simulink model "VC_v1p1"  (R2022b)
settings: Solver=VariableStepAuto  StartTime=0.0  StopTime=inf  FixedStep=1/100  MaxStep=ts  RelTol=1e-3
InitFcn:
  | init_car
  | init_par
values from neighbouring files (symbols this model uses):
  east0 = EWP(1)    [run_VC_bench.m]
  g = 9.81    [init_car.m]
  north0 = NWP(1)    [run_VC_bench.m]
  NUM_WP = length(NWP)    [run_VC_bench.m]
  psi0 = (pi/180)*HWP(1)    [run_VC_bench.m]
  ts = 1/fs    (= 0.01)    [init_car.m]
  vcg0 = 0    [run_VC_bench.m]
  WPT_MTX = [NWP,EWP,HWP,VWP,KWP,SWP]    [run_VC_bench.m]
undefined symbols (not defined in the file or in its folder): car, EWP, NWP, par, ZWP
libraries: simulink x9, matrix_library x6
(part 1 of 3)
Description:
  | This simulation was created by S. C. Southward to develop and validate control strategies for an autonomous vehicle modeled as a kinematic bicycle model.
settings Model: Creator=steve  LastModifiedBy=steve
settings SolverCC: AlgebraicLoopSolver=TrustRegion
settings DataIOCC: SaveOutput=off  SignalLogging=off  DSMLogging=off  SaveTime=off  ReturnWorkspaceOutputs=off
settings OptimizationCC: DefaultParameterBehavior=Inlined  UseDivisionForNetSlopeComputation=on  GainParamInheritBuiltInType=on  UseFloatMulNetSlope=on  InlineInvariantSignals=on  PassReuseOutputArgsAs=Individual arguments  ZeroExternalMemoryAtStartup=off  ZeroInternalMemoryAtStartup=off  NoFixptDivByZeroProtection=on  EfficientFloat2IntCast=on  LifeSpan=1  OptimizeBlockOrder=speed  DifferentSizesBufferReuse=on  EfficientTunableParamExpr=on
settings DebuggingCC: MaxConsecutiveZCsMsg=none  ParameterTunabilityLossMsg=error  UnderSpecifiedDataTypeMsg=warning  UnconnectedInputMsg=warning  UnconnectedOutputMsg=warning  UnconnectedLineMsg=warning  SFMachineParentedDataDiag=warning  UnderSpecifiedDimensionMsg=warning  ArithmeticOperatorsInVariantConditions=warning
settings HardwareCC: ProdBitPerLong=64  ProdLongLongMode=on  ProdHWDeviceType=Intel->x86-64 (Linux 64)
settings ModelReferenceCC: EnableRefExpFcnMdlSchedulingChecks=on
settings SFSimCC: SimUseLocalCustomCode=off  MATLABDynamicMemAlloc=off  CustomCodeUndefinedFunction=UseInterfaceOnly
settings RTWCC: Description=Embedded Coder  SystemTargetFile=ert.tlc  TemplateMakefile=ert_default_tmf  RTWUseLocalCustomCode=off  TargetLang=C++  DLArmComputeVersion=19.05
settings CodeAppCC: ForceParamTrailComments=on  IgnoreCustomStorageClasses=off  OperatorAnnotations=on  SimulinkDataObjDesc=on  SFDataObjDesc=on  CustomSymbolStrGlobalVar=rt$N$M  CustomSymbolStrType=$N$M  CustomSymbolStrFcn=$N$M$F  CustomSymbolStrMacro=$N$M  InsertBlockDesc=on
settings ERTTargetCC: TargetLangStandard=C++03 (ISO)  GenerateSampleERTMain=on  IncludeMdlTerminateFcn=off  CombineSignalStateStructs=on  CodeInterfacePackaging=C++ class  SupportComplex=off  SupportNonInlinedSFcns=on  InlinedParameterPlacement=NonHierarchical  RootIOFormat=Structure reference  ERTCustomFileTemplate=example_file_process.tlc  ERTFilePackagingFormat=CompactWithDataFile

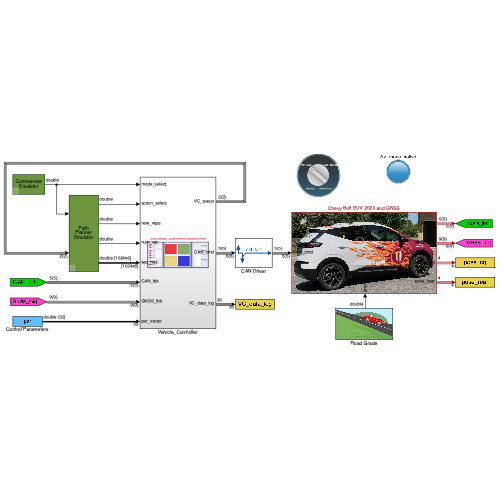
[thumbnail: Simulink's stored preview of the top-level diagram]
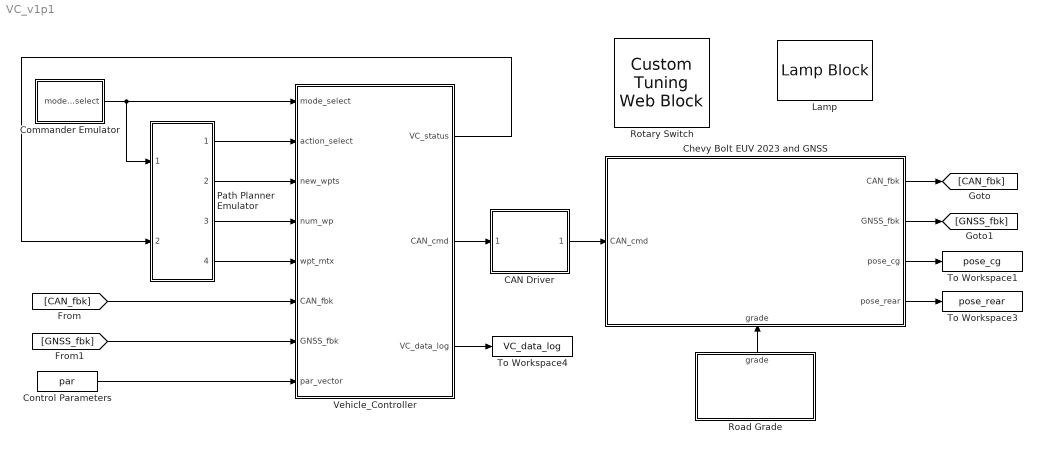
== system VC_v1p1 ==
  CAN Driver : Subsystem
      mask Display: image('$imagefile'); % Use "Edit Image" on toolstrip to change.
  Chevy Bolt EUV 2023 and GNSS : Subsystem
      settings: PortSchema="{\"entries\":[{\"content\":{\"sides\":[{\"content\":{\"connectorIds\":[\"In1\"]},\"type\":\"ConnectorPlacement.EquallySpacedRectSide\",\"uuid\":\"214ac55f-e1ad-4aeb-894e-d0c732f6c7ee\"},{\"content\":{\"connectorIds\":[\"Out1\",\"Out2\",\"Out3\",\"Out4\"],\"side\":\"RIGHT\"},\"type\":\"ConnectorPlacement.EquallySpacedRectSide\",\"uuid\":\"96b26d7b-3219-4372-aec8-5812d174b28b\"},{\"content\":{\"connectorIds\":[],\"side\":\"TOP\"},\"type\":\"ConnectorPlacement.EquallySpacedRectSide\",\"uuid\":\"1264bf6a-3e04-4574-8398-8e873a97a666\"},{\"content\":{\"connectorIds\":[\"In2\"],\"side\":\"BOTTOM\"},\"type\":\"ConnectorPlacement.EquallySpacedRectSide\",\"uuid\":\"d9b028eb-d70e-44ed-81e4-9460dc761106\"}]},\"type\":\"ConnectorPlacement.EquallySpacedConnector\",\"uuid\":\"c4360da5-3195-43cb-bf9a-daa7ef28b28e\"}],\"packageUris\":[\"http://schema.mathworks.com/mf0/Connector/R2020b\"],\"version\":\"1.0\"}"
      mask Display: image('$imagefile'); % Use "Edit Image" on toolstrip to change.
  Commander Emulator : Subsystem
      mask Display: fprintf('Commander\nEmulator');
  Control Parameters : Constant  Value=par  SampleTime=ts
  Lamp : LampBlock
  Path Planner Emulator : Subsystem
      mask Display: fprintf('Path\nPlanner\nEmulator');
  Road Grade : Subsystem
      settings: PortSchema="{\"entries\":[{\"content\":{\"sides\":[{\"content\":{\"connectorIds\":[]},\"type\":\"ConnectorPlacement.EquallySpacedRectSide\",\"uuid\":\"7eade820-9aea-479f-bbe1-ec2238160034\"},{\"content\":{\"connectorIds\":[],\"side\":\"RIGHT\"},\"type\":\"ConnectorPlacement.EquallySpacedRectSide\",\"uuid\":\"4478e073-9b69-4ee8-bedd-aa799e149f9b\"},{\"content\":{\"connectorIds\":[\"Out1\"],\"side\":\"TOP\"},\"type\":\"ConnectorPlacement.EquallySpacedRectSide\",\"uuid\":\"a531a2af-fb7a-43d6-8f4e-3d919d89502a\"}]},\"type\":\"ConnectorPlacement.EquallySpacedConnector\",\"uuid\":\"31b98e99-7583-4dbb-9f8b-3eb6bbb70df0\"}],\"packageUris\":[\"http://schema.mathworks.com/mf0/Connector/R2020b\"],\"version\":\"1.0\"}"
      mask Display: image('$imagefile'); % Use "Edit Image" on toolstrip to change.
  Rotary Switch : CustomTuningWebBlock  LabelPosition=Hide  ShowInitialText=on  Configuration="{\"components\":[{\"name\":\"RotarySwitchComponent\",\"settings\":{\"arcAngle\":300,\"arcAngleOffset\":120,\"handle\":{\"size\":[150,150],\"src\":\"data:image\\/svg+xml;base64,PHN2ZyBpZD0iTGF5ZXJfMSIgZGF0YS1uYW1lPSJMYXllciAxIiB4bWxucz0iaHR0cDovL3d3dy53My5vcmcvMjAwMC9zdmciIHhtbG5zOnhsaW5rPSJodHRwOi8vd3d3LnczLm9yZy8xOTk5L3hsaW5rIiB2aWV3Qm94PSIwIDAgMTIxIDEyMSI+PGRlZnM+PHN0eWxlPi5jbHMtMXtmaWxsOnVybCgjbGluZWFyLWdyYWRpZW50KTt9LmNscy0yLC5jbHMtM3tmaWxsOiNkMWQxZDE7fS5jbHMtM3tzdHJva2U6I2I3YjdiNztzdHJva2UtbWl0ZXJsaW1pdDoxMDtzdHJva2Utd2lkdGg6MC4yNXB4O30uY2xzLTR7ZmlsbDojZjMwMDAwO30uY2xzLTV7ZmlsbDojZjIxNzY3O308L3N0eWxlPjxsaW5lYXJHcmFkaWVudCBpZD0ibGluZWFyLWdyYWRpZW50IiB4MT0iNjAuNSIgeTE9IjEyMC41IiB4Mj0iNjAuNSIgeTI9IjAuNSIgZ3JhZGllbnRVbml0cz0idXNlclNwYWNlT25Vc2UiPjxzdG9wIG9mZnNldD0iMCIgc3RvcC1jb2xvcj0iI2QxZDFkMSIvPjxzdG9wIG9mZnNldD0iMC4xIiBzdG9wLWNvbG9yPSIjY2VjZWNlIi8+PHN0b3Agb2Zmc2V0PSIwLjE5IiBzdG9wLWNvbG9yPSIjYzNjM2MzIi8+PHN0b3Agb2Zmc2V0PSIwLjI4IiBzdG9wLWNvbG9yPSIjYjFiMWIxIi8+PHN0b3Agb2Zmc2V0PSIwLjM2IiBzdG9wLWNvbG9yPSIjOTg5ODk4Ii8+PHN0b3Agb2Zmc2V0PSIwLjQ0IiBzdG9wLWNvbG9yPSIjNzg3ODc4Ii8+PHN0b3Agb2Zmc2V0PSIwLjQ2IiBzdG9wLWNvbG9yPSIjNmI2YjZiIi8+PHN0b3Agb2Zmc2V0PSIwLjU0IiBzdG9wLWNvbG9yPSIjNmI2YjZiIi8+PHN0b3Agb2Zmc2V0PSIwLjU2IiBzdG9wLWNvbG9yPSIjNzY3Njc2Ii8+PHN0b3Agb2Zmc2V0PSIwLjY0IiBzdG9wLWNvbG9yPSIjOTc5Nzk3Ii8+PHN0b3Agb2Zmc2V0PSIwLjcyIiBzdG9wLWNvbG9yPSIjYjBiMGIwIi8+PHN0b3Agb2Zmc2V0PSIwLjgxIiBzdG9wLWNvbG9yPSIjYzNjM2MzIi8+PHN0b3Agb2Zmc2V0PSIwLjkiIHN0b3AtY29sb3I9IiNjZGNkY2QiLz48c3RvcCBvZmZzZXQ9IjEiIHN0b3AtY29sb3I9IiNkMWQxZDEiLz48L2xpbmVhckdyYWRpZW50PjwvZGVmcz48Y2lyY2xlIGNsYXNzPSJjbHMtMSIgY3g9IjYwLjUiIGN5PSI2MC41IiByPSI2MCIvPjxwYXRoIGNsYXNzPSJjbHMtMiIgZD0iTTYwLjUsMUE1OS41LDU5LjUsMCwxLDEsMSw2MC41LDU5LjU3LDU5LjU3LDAsMCwxLDYwLjUsMW0wLTFBNjAuNSw2MC41LDAsMSwwLDEyMSw2MC41LDYwLjUsNjAuNSwwLDAsMCw2MC41LDBaIi8+PHJlY3QgY2xhc3M9ImNscy0zIiB4PSIwLjUiIHk9IjUxLjUiIHdpZHRoPSIxMjAiIGhlaWdodD0iMTgiIHJ4PSIzLjA0Ii8+PHJlY3QgY2xhc3M9ImNscy00IiB4PSI1Ljc1IiB5PSI1OC43NSIgd2lkdGg9IjE2IiBoZWlnaHQ9IjMiLz48cGF0aCBjbGFzcz0iY2xzLTUiIGQ9Ik0yMS4yNSw1OS4yNXYyaC0xNXYtMmgxNW0xLTFoLTE3djRoMTd2LTRaIi8+PC9zdmc+\"},\"handleOffset\":[0,0],\"handleOrientation\":180,\"handlePosition\":[0,0,1,1],\"handleSize\":{\"height\":0.5,\"width\":0.5},\"labelRadius\":0.36,\"position\":[0,0,1,1],\"states\":[{\"Label\":{\"color\":[0,0,0,1],\"icon\":{\"size\":[0,0],\"src\":[],\"srcOrientation\":\"Right\"},\"iconPlacement\":\"left\",\"opacity\":1,\"position\":[0.7345552884615385,0.6796274038461538],\"show\":true,\"text\":{\"content\":\"Manual\",\"font\":\"Helvetica\",\"fontSize\":24}},\"Value\":0},{\"Label\":{\"color\":[0,0,0,1],\"icon\":{\"size\":[0,0],\"src\":[],\"srcOrientation\":\"Right\"},\"iconPlacement\":\"left\",\"opacity\":1,\"position\":[0.35757211538461536,0.7603966346153846],\"show\":true,\"text\":{\"content\":\"Full Auto\",\"font\":\"Helvetica\",\"fontSize\":24}},\"Value\":1},{\"Label\":{\"color\":[0,0,0,1],\"icon\":{\"size\":[0,0],\"src\":[],\"srcOrientation\":\"Right\"},\"iconPlacement\":\"left\",\"opacity\":1,\"position\":[0.09603365384615385,0.46033653846153844],\"show\":true,\"text\":{\"content\":\"Auto Speed\",\"font\":\"Helvetica\",\"fontSize\":24}},\"Value\":2},{\"Label\":{\"color\":[0,0,0,1],\"icon\":{\"size\":[0,0],\"src\":[],\"srcOrientation\":\"Right\"},\"iconPlacement\":\"left\",\"opacity\":1,\"position\":[0.36532451923076925,0.1180889423076923],\"show\":true,\"text\":{\"content\":\"Auto Steer\",\"font\":\"Helvetica\",\"fontSize\":24}},\"Value\":3}],\"tickRadius\":0.32}},{\"name\":\"BackgroundImageComponent\",\"settings\":{\"image\":{\"size\":[155,150],\"src\":\"data:image\\/svg+xml;base64,PD94bWwgdmVyc2lvbj0iMS4wIiBlbmNvZGluZz0idXRmLTgiPz4NCjwhLS0gR2VuZXJhdG9yOiBBZG9iZSBJbGx1c3RyYXRvciAyNS4wLjAsIFNWRyBFeHBvcnQgUGx1Zy1JbiAuIFNWRyBWZXJzaW9uOiA2LjAwIEJ1aWxkIDApICAtLT4NCjxzdmcgdmVyc2lvbj0iMS4xIg0KCSBpZD0iTGF5ZXJfMl8xXyIgeG1sbnM6Y2M9Imh0dHA6Ly9jcmVhdGl2ZWNvbW1vbnMub3JnL25zIyIgeG1sbnM6ZGM9Imh0dHA6Ly9wdXJsLm9yZy9kYy9lbGVtZW50cy8xLjEvIiB4bWxuczppbmtzY2FwZT0iaHR0cDovL3d3dy5pbmtzY2FwZS5vcmcv ...(+4184 chars)\",\"srcOrientation\":\"Right\"},\"position\":[0,0,1,1],\"scaleMode\":\"0\"}},{\"name\":\"ForegroundImageComponent\",\"settings\":{\"image\":{\"size\":[0,0],\"src\":\"default\",\"srcOrientation\":[]},\"isForeground\":1,\"position\":[0,0,1,1],\"scaleMode\":\"0\"}}],\"settings\":{\"BindingType\":\"param\",\"backgroundColor\":[0,0,255,\"1\"],\"backgroundOffset\":1,\"fixedAspectRatio\":\"on\",\"image\":{\"size\":[150,150],\"src\":\"data:image\\/svg+xml;base64,PD94bWwgdmVyc2lvbj0iMS4wIiBlbmNvZGluZz0iVVRGLTgiIHN0YW5kYWxvbmU9Im5vIj8+CjwhLS0gR2VuZXJhdG9yOiBBZG9iZSBJbGx1c3RyYXRvciAxOS4yLjEsIFNWRyBFeHBvcnQgUGx1Zy1JbiAuIFNWRyBWZXJzaW9uOiA2LjAwIEJ1aWxkIDApICAtLT4KCjxzdmcKICAgeG1sbnM6ZGM9Imh0dHA6Ly9wdXJsLm9yZy9kYy9lbGVtZW50cy8xLjEvIgogICB4bWxuczpjYz0iaHR0cDovL2NyZWF0aXZlY29tbW9ucy5vcmcvbnMjIgogICB4bWxuczpyZGY9Imh0dHA6Ly93d3cudzMub3JnLzE5OTkvMDIvMjItcmRmLXN5bnRh ...(+9660 chars)\"},\"showBackgroundColor\":false,\"variant\":\"rotarySwitch\",\"version\":\"R2022b\"},\"type\":\"RotarySwitch\"}"
  To Workspace1 : ToWorkspace  VariableName=pose_cg  SampleTime=ts
  To Workspace3 : ToWorkspace  VariableName=pose_rear  SampleTime=ts
  To Workspace4 : ToWorkspace  VariableName=VC_data_log  SampleTime=ts
  Vehicle_Controller : Subsystem
  wires:
  Vehicle_Controller/2(CAN_cmd) -> CAN Driver/1(CAN_cmd)
  Road Grade/1(grade) -> Chevy Bolt EUV 2023 and GNSS/2(grade)
  Chevy Bolt EUV 2023 and GNSS/1(CAN_fbk) -> [CAN_fbk]
  Chevy Bolt EUV 2023 and GNSS/4(pose_rear) -> To Workspace3/1
  Chevy Bolt EUV 2023 and GNSS/3(pose_cg) -> To Workspace1/1
  Chevy Bolt EUV 2023 and GNSS/2(GNSS_fbk) -> [GNSS_fbk]
  [CAN_fbk] -> Vehicle_Controller/6(CAN_fbk)
  [GNSS_fbk] -> Vehicle_Controller/7(GNSS_fbk)
  Vehicle_Controller/3(VC_data_log) -> To Workspace4/1
  CAN Driver/1(CAN_cmd_out) -> Chevy Bolt EUV 2023 and GNSS/1(CAN_cmd)
  Control Parameters/1 -> Vehicle_Controller/8(par_vector)
  Vehicle_Controller/1(VC_status) -> Path Planner Emulator/2(VC_status)
  Commander Emulator/1(mode_select) -> Vehicle_Controller/1(mode_select), Path Planner Emulator/1(mode_select)
  Path Planner Emulator/1(action_select) -> Vehicle_Controller/2(action_select)
  Path Planner Emulator/4(wpt_mtx) -> Vehicle_Controller/5(wpt_mtx)
  Path Planner Emulator/3(num_wp) -> Vehicle_Controller/4(num_wp)
  Path Planner Emulator/2(new_wpts) -> Vehicle_Controller/3(new_wpts)

== system VC_v1p1/CAN Driver ==
  note: This code block is the set of CAN driver functions that convert command signals to
      | appropriate 8-byte CAN messages.
  CAN_cmd : Inport
  Bus Creator : BusCreator  Inputs=5
  Bus Selector : BusSelector  OutputSignals=AV_start_request,mode_select,torque_cmd,brake_cmd,steer_cmd,signal_cmd
  MATLAB Function : MATLAB Function  TreatAsAtomicUnit=on
  CAN_cmd_out : Outport
  wires:
  CAN_cmd/1 -> Bus Selector/1
  Bus Creator/1 -> CAN_cmd_out/1
  Bus Selector/1 -> MATLAB Function/1(AV_start_request)  "<AV_start_request>"
  Bus Selector/2 -> MATLAB Function/2(mode_select)  "<mode_select>"
  Bus Selector/3 -> MATLAB Function/3(torque_in)  "<torque_cmd>"
  Bus Selector/4 -> MATLAB Function/4(brake_in)  "<brake_cmd>"
  Bus Selector/5 -> MATLAB Function/5(steer_in)  "<steer_cmd>"
  Bus Selector/6 -> MATLAB Function/6(signal_in)  "<signal_cmd>"
  MATLAB Function/2(torque_cmd) -> Bus Creator/2  "torque_cmd"
  MATLAB Function/3(brake_cmd) -> Bus Creator/3  "brake_cmd"
  MATLAB Function/4(steer_cmd) -> Bus Creator/4  "steer_cmd"
  MATLAB Function/5(gear_cmd) -> Bus Creator/5  "gear_cmd"
  MATLAB Function/1(AV_mode_active) -> Bus Creator/1  "AV_mode_active"

== system VC_v1p1/Chevy Bolt EUV 2023 and GNSS ==
  CAN_cmd : Inport
  grade : Inport  Port=2
  Bus Selector : BusSelector  OutputSignals=vcg (m/s)
  GNSS measurement : Subsystem
  engine-steer-brake and inertial dynamics : Subsystem
  kinematic Bicycle model : Subsystem
      mask Display: image('$imagefile'); % Use "Edit Image" on toolstrip to change.
  CAN_fbk : Outport  VectorParamsAs1DForOutWhenUnconnected=off
  GNSS_fbk : Outport  Port=2  VectorParamsAs1DForOutWhenUnconnected=off
  pose_cg : Outport  Port=3  VectorParamsAs1DForOutWhenUnconnected=off
  pose_rear : Outport  Port=4  VectorParamsAs1DForOutWhenUnconnected=off
  wires:
  engine-steer-brake and inertial dynamics/2(delta (rad)) -> kinematic Bicycle model/1(delta (rad))  "delta (rad)"
  engine-steer-brake and inertial dynamics/1(CAN_fbk) -> CAN_fbk/1
  grade/1 -> engine-steer-brake and inertial dynamics/2(grade (rad))
  kinematic Bicycle model/2(pose_rear) -> pose_rear/1, GNSS measurement/2(pose_rear)
  GNSS measurement/1(GNSS_fbk) -> GNSS_fbk/1
  CAN_cmd/1 -> engine-steer-brake and inertial dynamics/1(CAN_cmd)
  engine-steer-brake and inertial dynamics/3(IMU_fbk) -> Bus Selector/1, GNSS measurement/4(IMU_fbk)
  Bus Selector/1 -> kinematic Bicycle model/2(vcg (m/s))  "<vcg (m/s)>"
  kinematic Bicycle model/3(kappa (1/m)) -> GNSS measurement/3(kappa (1/m))  "kappa (1/m)"
  kinematic Bicycle model/1(pose_cg) -> pose_cg/1, GNSS measurement/1(pose_cg)

== system VC_v1p1/Commander Emulator ==
  note: mode_select
      | 0 = manual
      | 1 = full autonomous
      | 2 = autonomous speed
      | 3 = autonomous steer
  Mode Selection : Constant  SampleTime=ts
  Sample Delay : UnitDelay  SampleTime=ts  HasFrameUpgradeWarning=on
  mode_select : Outport
  wires:
  Mode Selection/1 -> Sample Delay/1
  Sample Delay/1 -> mode_select/1

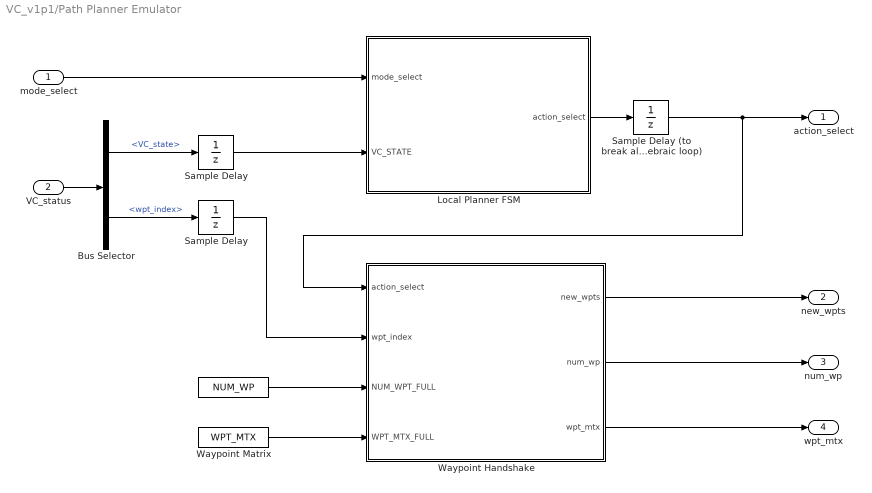
== system VC_v1p1/Path Planner Emulator ==
  mode_select : Inport
  VC_status : Inport  Port=2
  "   " : Constant  Value=NUM_WP  SampleTime=ts
  Bus Selector : BusSelector  OutputSignals=VC_state,wpt_index
  Local Planner FSM : Stateflow chart  TreatAsAtomicUnit=on  SystemSampleTime=1/100
  Sample Delay : UnitDelay  SampleTime=ts  HasFrameUpgradeWarning=on
  Sample Delay (to break algebraic loop) : UnitDelay  SampleTime=ts  HasFrameUpgradeWarning=on
  "Sample Delay " : UnitDelay  SampleTime=ts  HasFrameUpgradeWarning=on
  Waypoint Handshake : MATLAB Function  TreatAsAtomicUnit=on
  Waypoint Matrix : Constant  Value=WPT_MTX  SampleTime=ts
  action_select : Outport
  new_wpts : Outport  Port=2
  num_wp : Outport  Port=3
  wpt_mtx : Outport  Port=4
  wires:
  VC_status/1 -> Bus Selector/1
  Local Planner FSM/1(action_select) -> Sample Delay (to break algebraic loop)/1
  Bus Selector/1 -> Sample Delay/1  "<VC_state>"
  mode_select/1 -> Local Planner FSM/1(mode_select)
  Sample Delay/1 -> Local Planner FSM/2(VC_STATE)
  Sample Delay (to break algebraic loop)/1 -> Waypoint Handshake/1(action_select), action_select/1
  Waypoint Handshake/3(wpt_mtx) -> wpt_mtx/1
  Waypoint Handshake/2(num_wp) -> num_wp/1
  Waypoint Handshake/1(new_wpts) -> new_wpts/1
  "   "/1 -> Waypoint Handshake/3(NUM_WPT_FULL)
  Waypoint Matrix/1 -> Waypoint Handshake/4(WPT_MTX_FULL)
  Bus Selector/2 -> "Sample Delay "/1  "<wpt_index>"
  "Sample Delay "/1 -> Waypoint Handshake/2(wpt_index)

== system VC_v1p1/Road Grade ==
  MATLAB Function : MATLAB Function  TreatAsAtomicUnit=on
  easting waypoints : Constant  Value=EWP  SampleTime=ts
  elevation waypoints : Constant  Value=ZWP  SampleTime=ts
  northing waypoints : Constant  Value=NWP  SampleTime=ts
  grade : Outport
  wires:
  MATLAB Function/1(grade_rad) -> grade/1
  [wpt_index] -> MATLAB Function/1(wpt_index)
  elevation waypoints/1 -> MATLAB Function/4(ZWP)  "grade"
  northing waypoints/1 -> MATLAB Function/2(NWP)  "grade"
  easting waypoints/1 -> MATLAB Function/3(EWP)  "grade"

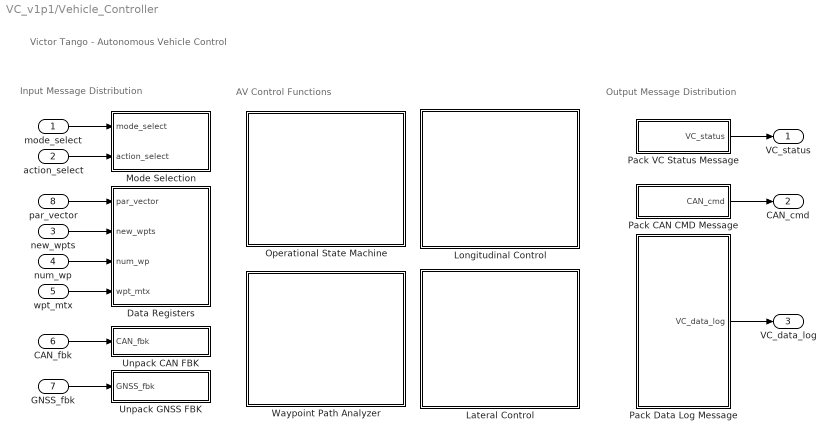
== system VC_v1p1/Vehicle_Controller ==
  note: Victor Tango - Autonomous Vehicle Control
  note: AV Control Functions
  note: Output Message Distribution
  note: Input Message Distribution
  mode_select : Inport
  action_select : Inport  Port=2
  new_wpts : Inport  Port=3
  num_wp : Inport  Port=4
  wpt_mtx : Inport  Port=5
  CAN_fbk : Inport  Port=6
  GNSS_fbk : Inport  Port=7
  par_vector : Inport  Port=8
  Data Registers : Subsystem
      mask Display: image('$imagefile'); % Use "Edit Image" on toolstrip to change.
  Lateral Control : Subsystem
      mask Display: image('$imagefile'); % Use "Edit Image" on toolstrip to change.
  Longitudinal Control : Subsystem
      mask Display: image('$imagefile'); % Use "Edit Image" on toolstrip to change.
  Mode Selection : Subsystem
      mask Display: image('$imagefile'); % Use "Edit Image" on toolstrip to change.
  Operational State Machine : Subsystem
      mask Display: image('$imagefile'); % Use "Edit Image" on toolstrip to change.
  Pack CAN CMD Message : Subsystem
      mask Display: image('$imagefile'); % Use "Edit Image" on toolstrip to change.
  Pack Data Log Message : Subsystem
      mask Display: image('$imagefile'); % Use "Edit Image" on toolstrip to change.
  Pack VC Status Message : Subsystem
      mask Display: image('$imagefile'); % Use "Edit Image" on toolstrip to change.
  Unpack CAN FBK : Subsystem
      mask Display: image('$imagefile'); % Use "Edit Image" on toolstrip to change.
  Unpack GNSS FBK : Subsystem
      mask Display: image('$imagefile'); % Use "Edit Image" on toolstrip to change.
  Waypoint Path Analyzer : Subsystem
      mask Display: image('$imagefile'); % Use "Edit Image" on toolstrip to change.
  VC_status : Outport
  CAN_cmd : Outport  Port=2
  VC_data_log : Outport  Port=3
  wires:
  Pack Data Log Message/1(VC_data_log) -> VC_data_log/1
  Pack CAN CMD Message/1(CAN_cmd) -> CAN_cmd/1
  CAN_fbk/1 -> Unpack CAN FBK/1(CAN_fbk)
  GNSS_fbk/1 -> Unpack GNSS FBK/1(GNSS_fbk)
  mode_select/1 -> Mode Selection/1(mode_select)
  action_select/1 -> Mode Selection/2(action_select)
  par_vector/1 -> Data Registers/1(par_vector)
  new_wpts/1 -> Data Registers/2(new_wpts)
  wpt_mtx/1 -> Data Registers/4(wpt_mtx)
  Pack VC Status Message/1(VC_status) -> VC_status/1
  num_wp/1 -> Data Registers/3(num_wp)

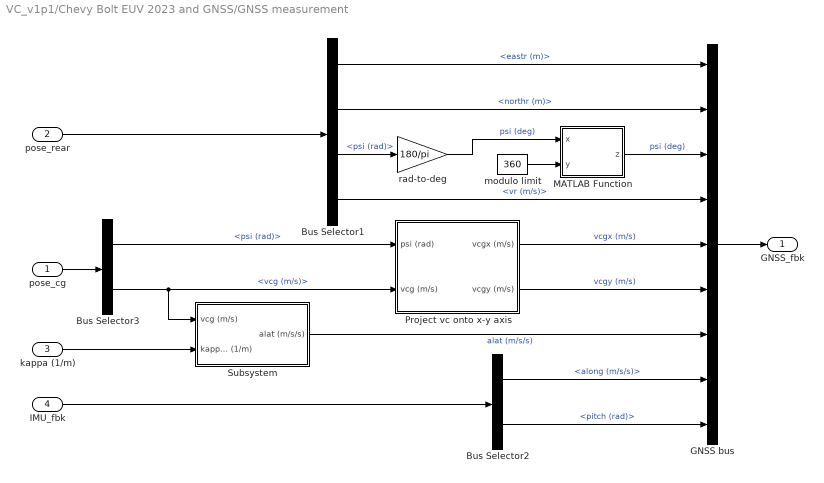
== system VC_v1p1/Chevy Bolt EUV 2023 and GNSS/GNSS measurement ==
  pose_cg : Inport
  pose_rear : Inport  Port=2
  kappa (1/m) : Inport  Port=3
  IMU_fbk : Inport  Port=4
  Bus Selector1 : BusSelector  OutputSignals=eastr (m),northr (m),psi (rad),vr (m/s)
  Bus Selector2 : BusSelector  OutputSignals=along (m/s/s),pitch (rad)
  Bus Selector3 : BusSelector  OutputSignals=psi (rad),vcg (m/s)
  GNSS bus : BusCreator  Inputs=9
  MATLAB Function : MATLAB Function  TreatAsAtomicUnit=on
  Project vc onto x-y axis : Subsystem
  Subsystem : Subsystem
  modulo limit : Constant  Value=360
  rad-to-deg : Gain  Gain=180/pi
  GNSS_fbk : Outport
  wires:
  GNSS bus/1 -> GNSS_fbk/1
  rad-to-deg/1 -> MATLAB Function/1(x)  "psi (deg)"
  pose_rear/1 -> Bus Selector1/1
  IMU_fbk/1 -> Bus Selector2/1
  Bus Selector1/1 -> GNSS bus/1  "<eastr (m)>"
  Bus Selector1/2 -> GNSS bus/2  "<northr (m)>"
  Bus Selector1/3 -> rad-to-deg/1  "<psi (rad)>"
  Bus Selector1/4 -> GNSS bus/4  "<vr (m/s)>"
  Bus Selector2/1 -> GNSS bus/8  "<along (m/s/s)>"
  Bus Selector2/2 -> GNSS bus/9  "<pitch (rad)>"
  Project vc onto x-y axis/1(vcgx (m/s)) -> GNSS bus/5  "vcgx (m/s)"
  Project vc onto x-y axis/2(vcgy (m/s)) -> GNSS bus/6  "vcgy (m/s)"
  Subsystem/1(alat (m/s/s)) -> GNSS bus/7  "alat (m/s/s)"
  pose_cg/1 -> Bus Selector3/1
  Bus Selector3/2 -> Subsystem/1(vcg (m/s)), Project vc onto x-y axis/2(vcg (m/s))  "<vcg (m/s)>"
  kappa (1/m)/1 -> Subsystem/2(kappa (1/m))
  Bus Selector3/1 -> Project vc onto x-y axis/1(psi (rad))  "<psi (rad)>"
  MATLAB Function/1(z) -> GNSS bus/3  "psi (deg)"
  modulo limit/1 -> MATLAB Function/2(y)

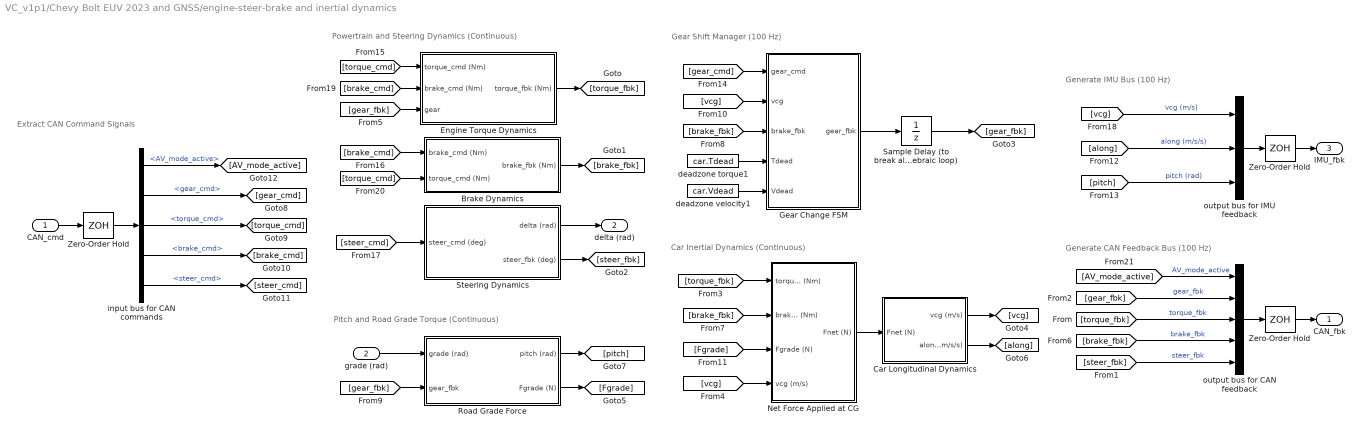
== system VC_v1p1/Chevy Bolt EUV 2023 and GNSS/engine-steer-brake and inertial dynamics ==
  note: Generate CAN Feedback Bus (100 Hz)
  note: Powertrain and Steering Dynamics (Continuous)
  note: Pitch and Road Grade Torque (Continuous)
  note: Generate IMU Bus (100 Hz)
  note: Extract CAN Command Signals
  note: Car Inertial Dynamics (Continuous)
  note: Gear Shift Manager (100 Hz)
  CAN_cmd : Inport
  grade (rad) : Inport  Port=2
  Brake Dynamics : Subsystem
  Car Longitudinal Dynamics : Subsystem
  Engine Torque Dynamics : Subsystem
  Gear Change FSM : Stateflow chart  TreatAsAtomicUnit=on  SystemSampleTime=ts
  Net Force Applied at CG : Subsystem
  Road Grade Force : Subsystem
  Sample Delay (to break algebraic loop) : UnitDelay  SampleTime=ts  HasFrameUpgradeWarning=on
  Steering Dynamics : Subsystem
  Zero-Order Hold : ZeroOrderHold  SampleTime=ts
  "Zero-Order Hold " : ZeroOrderHold  SampleTime=ts
  "Zero-Order Hold  " : ZeroOrderHold  SampleTime=ts
  deadzone torque1 : Constant  Value=car.Tdead  SampleTime=ts
  deadzone velocity1 : Constant  Value=car.Vdead  SampleTime=ts
  input bus for CAN commands : BusSelector  OutputSignals=AV_mode_active,gear_cmd,torque_cmd,brake_cmd,steer_cmd
  output bus for IMU feedback : BusCreator  Inputs=3
  output bus for CAN feedback : BusCreator  Inputs=5
  CAN_fbk : Outport  VectorParamsAs1DForOutWhenUnconnected=off
  delta (rad) : Outport  Port=2  VectorParamsAs1DForOutWhenUnconnected=off
  IMU_fbk : Outport  Port=3  VectorParamsAs1DForOutWhenUnconnected=off
  wires:
  deadzone velocity1/1 -> Gear Change FSM/5(Vdead)
  Steering Dynamics/1(delta (rad)) -> delta (rad)/1
  deadzone torque1/1 -> Gear Change FSM/4(Tdead)
  input bus for CAN commands/3 -> [torque_cmd]  "<torque_cmd>"
  Road Grade Force/2(Fgrade (N)) -> [Fgrade]
  [torque_fbk] -> output bus for CAN feedback/3  "torque_fbk"
  output bus for CAN feedback/1 -> "Zero-Order Hold  "/1
  CAN_cmd/1 -> Zero-Order Hold/1
  Brake Dynamics/1(brake_fbk (Nm)) -> [brake_fbk]
  [vcg] -> Gear Change FSM/2(vcg)
  [torque_cmd] -> Engine Torque Dynamics/1(torque_cmd (Nm))
  [brake_cmd] -> Brake Dynamics/1(brake_cmd (Nm))
  input bus for CAN commands/4 -> [brake_cmd]  "<brake_cmd>"
  [brake_fbk] -> Gear Change FSM/3(brake_fbk)
  [gear_fbk] -> Engine Torque Dynamics/3(gear)
  [torque_fbk] -> Net Force Applied at CG/1(torque_fbk (Nm))
  [gear_fbk] -> output bus for CAN feedback/2  "gear_fbk"
  [vcg] -> output bus for IMU feedback/1  "vcg (m/s)"
  [gear_cmd] -> Gear Change FSM/1(gear_cmd)
  [along] -> output bus for IMU feedback/2  "along (m/s/s)"
  [Fgrade] -> Net Force Applied at CG/3(Fgrade (N))
  output bus for IMU feedback/1 -> "Zero-Order Hold "/1
  Gear Change FSM/1(gear_fbk) -> Sample Delay (to break algebraic loop)/1
  Engine Torque Dynamics/1(torque_fbk (Nm)) -> [torque_fbk]
  input bus for CAN commands/2 -> [gear_cmd]  "<gear_cmd>"
  [steer_fbk] -> output bus for CAN feedback/5  "steer_fbk"
  Car Longitudinal Dynamics/1(vcg (m/s)) -> [vcg]
  Car Longitudinal Dynamics/2(along  (m/s/s)) -> [along]
  Steering Dynamics/2(steer_fbk (deg)) -> [steer_fbk]
  [brake_fbk] -> output bus for CAN feedback/4  "brake_fbk"
  Road Grade Force/1(pitch (rad)) -> [pitch]
  input bus for CAN commands/5 -> [steer_cmd]  "<steer_cmd>"
  Net Force Applied at CG/1(Fnet (N)) -> Car Longitudinal Dynamics/1(Fnet (N))
  [steer_cmd] -> Steering Dynamics/1(steer_cmd (deg))
  [pitch] -> output bus for IMU feedback/3  "pitch (rad)"
  grade (rad)/1 -> Road Grade Force/1(grade (rad))
  [brake_fbk] -> Net Force Applied at CG/2(brake_fbk (Nm))
  Zero-Order Hold/1 -> input bus for CAN commands/1
  Sample Delay (to break algebraic loop)/1 -> [gear_fbk]
  "Zero-Order Hold "/1 -> IMU_fbk/1
  "Zero-Order Hold  "/1 -> CAN_fbk/1
  [vcg] -> Net Force Applied at CG/4(vcg (m/s))
  [gear_fbk] -> Road Grade Force/2(gear_fbk)
  [brake_cmd] -> Engine Torque Dynamics/2(brake_cmd (Nm))
  [torque_cmd] -> Brake Dynamics/2(torque_cmd (Nm))
  input bus for CAN commands/1 -> [AV_mode_active]  "<AV_mode_active>"
  [AV_mode_active] -> output bus for CAN feedback/1  "AV_mode_active"

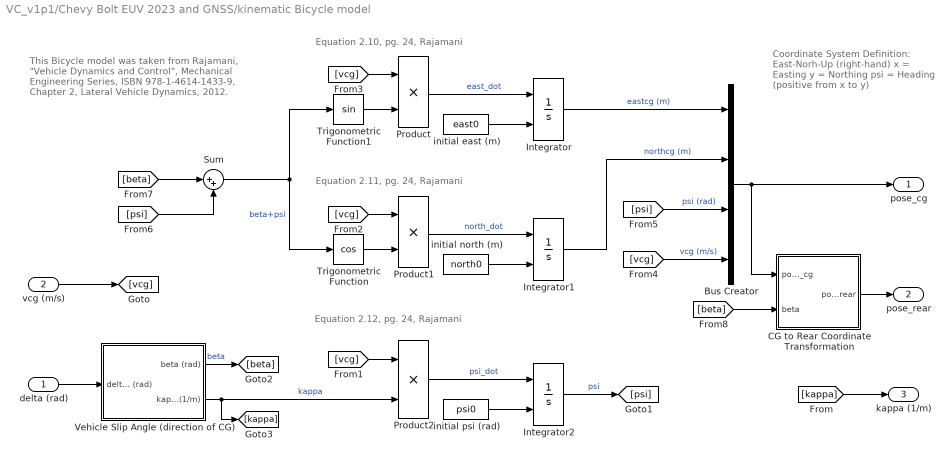
== system VC_v1p1/Chevy Bolt EUV 2023 and GNSS/kinematic Bicycle model ==
  note: Coordinate System Definition:
      | East-Norh-Up (right-hand)
      | x = Easting
      | y = Northing
      | psi = Heading (positive from x to y)
  note: Equation 2.10, pg. 24, Rajamani
  note: Equation 2.11, pg. 24, Rajamani
  note: Equation 2.12, pg. 24, Rajamani
  note: This Bicycle model was taken from Rajamani, "Vehicle Dynamics and Control", Mechanical Engineering Series, ISBN 978-1-4614-1433-9, Chapter 2, Lateral Vehicle Dynamics, 2012.
  delta (rad) : Inport
  vcg (m/s) : Inport  Port=2
  Bus Creator : BusCreator  Inputs=4
  CG to Rear Coordinate Transformation : Subsystem
  Integrator : Integrator  InitialConditionSource=external
  Integrator1 : Integrator  InitialConditionSource=external
  Integrator2 : Integrator  InitialConditionSource=external
  Product : Product
  Product1 : Product
  Product2 : Product
  Sum : Sum  Inputs=|++
  Trigonometric Function : Trigonometry  Operator=cos  OutputSignalType=real
  Trigonometric Function1 : Trigonometry  OutputSignalType=real
  Vehicle Slip Angle (direction of CG) : Subsystem
  initial east (m) : Constant  Value=east0
  initial north (m) : Constant  Value=north0
  initial psi (rad) : Constant  Value=psi0
  pose_cg : Outport  VectorParamsAs1DForOutWhenUnconnected=off
  pose_rear : Outport  Port=2  VectorParamsAs1DForOutWhenUnconnected=off
  kappa (1/m) : Outport  Port=3  VectorParamsAs1DForOutWhenUnconnected=off
  wires:
  Trigonometric Function1/1 -> Product/2
  Sum/1 -> Trigonometric Function1/1, Trigonometric Function/1  "beta+psi"
  vcg (m/s)/1 -> [vcg]
  Trigonometric Function/1 -> Product1/2
  Product1/1 -> Integrator1/1  "north_dot"
  Product2/1 -> Integrator2/1  "psi_dot"
  Product/1 -> Integrator/1  "east_dot"
  initial east (m)/1 -> Integrator/2
  initial north (m)/1 -> Integrator1/2
  initial psi (rad)/1 -> Integrator2/2
  [vcg] -> Product2/1
  [vcg] -> Product1/1
  [vcg] -> Product/1
  Bus Creator/1 -> CG to Rear Coordinate Transformation/1(pose_cg), pose_cg/1
  Integrator2/1 -> [psi]  "psi"
  Vehicle Slip Angle (direction of CG)/1(beta (rad)) -> [beta]  "beta"
  delta (rad)/1 -> Vehicle Slip Angle (direction of CG)/1(delta (rad))
  Vehicle Slip Angle (direction of CG)/2(kappa (1/m)) -> [kappa], Product2/2  "kappa"
  [psi] -> Sum/2
  [psi] -> Bus Creator/3  "psi (rad)"
  [vcg] -> Bus Creator/4  "vcg (m/s)"
  Integrator/1 -> Bus Creator/1  "eastcg (m)"
  Integrator1/1 -> Bus Creator/2  "northcg (m)"
  [beta] -> Sum/1
  CG to Rear Coordinate Transformation/1(pose_rear) -> pose_rear/1
  [beta] -> CG to Rear Coordinate Transformation/2(beta)
  [kappa] -> kappa (1/m)/1

== system VC_v1p1/Vehicle_Controller/Data Registers ==
  par_vector : Inport
  new_wpts : Inport  Port=2
  num_wp : Inport  Port=3
  wpt_mtx : Inport  Port=4
  load new parameter vector : Subsystem
      mask Display: image('$imagefile'); % Use "Edit Image" on toolstrip to change.
  load new waypoint matrix : Subsystem
      mask Display: image('$imagefile'); % Use "Edit Image" on toolstrip to change.
  tag scope: WPT_BUS=global, par_bus=global, wpt_status_change=global
  wires:
  par_vector/1 -> load new parameter vector/2(par_vector)
  [mode_select] -> load new parameter vector/1(mode_select)
  load new parameter vector/1(par_bus_out) -> [par_bus]  "par_bus"
  load new waypoint matrix/2(wpt_bus_out) -> [WPT_BUS]  "wpt_bus"
  load new waypoint matrix/1(wpt_status_change) -> [wpt_status_change]  "wpt_status_change"
  new_wpts/1 -> load new waypoint matrix/1(new_wpts)
  wpt_mtx/1 -> load new waypoint matrix/3(wpt_mtx)
  num_wp/1 -> load new waypoint matrix/2(num_wp)

== system VC_v1p1/Vehicle_Controller/Lateral Control ==
  Lateral Controller : Subsystem
  tag scope: kdes=global, kpdes=global, steer_cmd=global
  wires:
  [steer_mode] -> Lateral Controller/1(steer_mode)
  [psi] -> Lateral Controller/8(psi)
  [par_bus] -> Lateral Controller/9(par)
  Lateral Controller/1(steer_cmd) -> [steer_cmd]
  [east_target] -> Lateral Controller/5(east_target)
  [north_target] -> Lateral Controller/4(north_target)
  [vcar] -> Lateral Controller/7(vcar)
  [northr] -> Lateral Controller/3(northr)
  [steer_fbk] -> Lateral Controller/6(steer_fbk)
  [eastr] -> Lateral Controller/2(eastr)
  Lateral Controller/2(kpdes) -> [kpdes]
  Lateral Controller/3(kdes) -> [kdes]

== system VC_v1p1/Vehicle_Controller/Longitudinal Control ==
  Longitudinal Controller : Subsystem
  tag scope: brake_cmd=global, car_is_stopped=global, torque_cmd=global, vdes=global
  wires:
  [pitch] -> Longitudinal Controller/6(pitch)
  Longitudinal Controller/1(torque_cmd) -> [torque_cmd]
  [alat] -> Longitudinal Controller/4(alat)
  [vcar] -> Longitudinal Controller/3(vcar)
  [along] -> Longitudinal Controller/5(along)
  Longitudinal Controller/3(vdes) -> [vdes]
  Longitudinal Controller/2(brake_cmd) -> [brake_cmd]
  [vref] -> Longitudinal Controller/2(vref)
  [par_bus] -> Longitudinal Controller/7(par)
  [speed_mode] -> Longitudinal Controller/1(speed_mode)
  Longitudinal Controller/4(car_is_stopped) -> [car_is_stopped]

== system VC_v1p1/Vehicle_Controller/Mode Selection ==
  note: mode_select is an input from commander
  note: mode_select
      | 0 = manual
      | 1 = full autonomous
      | 2 = autonomous speed
      | 3 = autonomous steer
  note: action_select
      | 0 = enter manual mode
      | 1 = enter autonomous mode
      | 2 = enter run_hot mode
  note: action_select is an input from local planner
  mode_select : Inport
  action_select : Inport  Port=2
  tag scope: action_select=global, mode_select=global
  wires:
  mode_select/1 -> [mode_select]  "mode_select"
  action_select/1 -> [action_select]  "action_select"

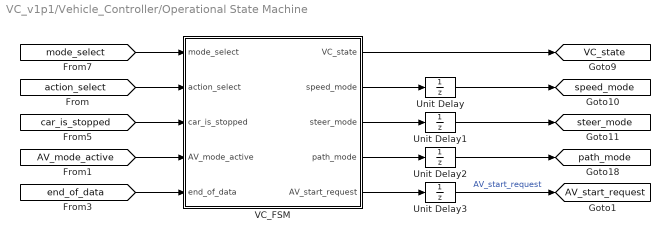
== system VC_v1p1/Vehicle_Controller/Operational State Machine ==
  Unit Delay{,1..3} (4 alike) : UnitDelay  SampleTime=ts  HasFrameUpgradeWarning=on
  VC_FSM : Stateflow chart  TreatAsAtomicUnit=on  SystemSampleTime=ts
  tag scope: AV_start_request=global, VC_state=global, path_mode=global, speed_mode=global, steer_mode=global
  wires:
  VC_FSM/2(speed_mode) -> Unit Delay/1
  VC_FSM/3(steer_mode) -> Unit Delay1/1
  VC_FSM/4(path_mode) -> Unit Delay2/1
  VC_FSM/1(VC_state) -> [VC_state]
  [action_select] -> VC_FSM/2(action_select)
  [mode_select] -> VC_FSM/1(mode_select)
  [car_is_stopped] -> VC_FSM/3(car_is_stopped)
  VC_FSM/5(AV_start_request) -> Unit Delay3/1
  [AV_mode_active] -> VC_FSM/4(AV_mode_active)
  Unit Delay/1 -> [speed_mode]
  Unit Delay1/1 -> [steer_mode]
  Unit Delay2/1 -> [path_mode]
  Unit Delay3/1 -> [AV_start_request]  "AV_start_request"
  [end_of_data] -> VC_FSM/5(end_of_data)

== system VC_v1p1/Vehicle_Controller/Pack CAN CMD Message ==
  output bus for CAN commands : BusCreator  Inputs=6
  CAN_cmd : Outport
  wires:
  [AV_start_request] -> output bus for CAN commands/1
  [torque_cmd] -> output bus for CAN commands/3
  [signal_cmd] -> output bus for CAN commands/6
  [brake_cmd] -> output bus for CAN commands/4
  output bus for CAN commands/1 -> CAN_cmd/1
  [steer_cmd] -> output bus for CAN commands/5
  [mode_select] -> output bus for CAN commands/2

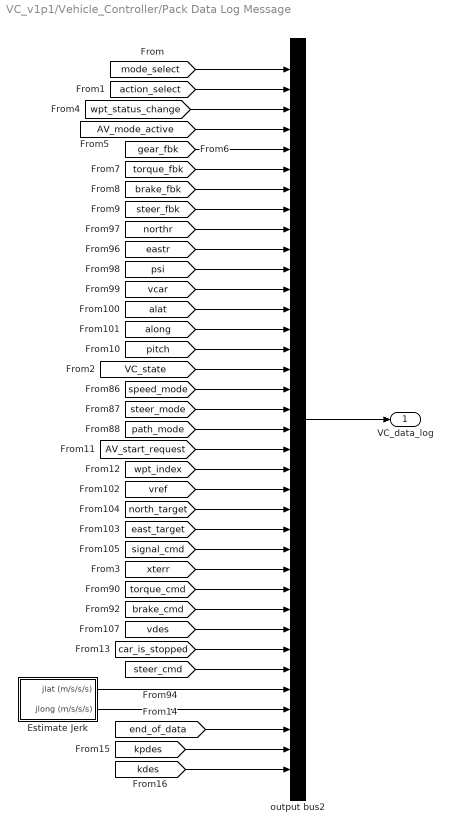
== system VC_v1p1/Vehicle_Controller/Pack Data Log Message ==
  Estimate Jerk : Subsystem
  output bus2 : BusCreator  Inputs=36
  VC_data_log : Outport
  wires:
  [mode_select] -> output bus2/1
  [action_select] -> output bus2/2
  [AV_mode_active] -> output bus2/4
  [gear_fbk] -> output bus2/5
  [torque_fbk] -> output bus2/6
  [brake_fbk] -> output bus2/7
  [steer_fbk] -> output bus2/8
  [northr] -> output bus2/9
  [eastr] -> output bus2/10
  [psi] -> output bus2/11
  [vcar] -> output bus2/12
  [alat] -> output bus2/13
  [along] -> output bus2/14
  [pitch] -> output bus2/15
  [VC_state] -> output bus2/16
  [speed_mode] -> output bus2/17
  [steer_mode] -> output bus2/18
  [path_mode] -> output bus2/19
  [AV_start_request] -> output bus2/20
  [wpt_index] -> output bus2/21
  [vref] -> output bus2/22
  [north_target] -> output bus2/23
  [east_target] -> output bus2/24
  [signal_cmd] -> output bus2/25
  [xterr] -> output bus2/26
  [torque_cmd] -> output bus2/27
  [brake_cmd] -> output bus2/28
  [vdes] -> output bus2/29
  [car_is_stopped] -> output bus2/30
  [steer_cmd] -> output bus2/31
  Estimate Jerk/1(jlat (m/s/s/s)) -> output bus2/32
  Estimate Jerk/2(jlong (m/s/s/s)) -> output bus2/33
  output bus2/1 -> VC_data_log/1
  [wpt_status_change] -> output bus2/3
  [end_of_data] -> output bus2/34
  [kpdes] -> output bus2/35
  [kdes] -> output bus2/36

== system VC_v1p1/Vehicle_Controller/Pack VC Status Message ==
  Bus Creator : BusCreator  Inputs=2
  VC_status : Outport
  wires:
  Bus Creator/1 -> VC_status/1
  [VC_state] -> Bus Creator/1
  [wpt_index] -> Bus Creator/2

== system VC_v1p1/Vehicle_Controller/Unpack CAN FBK ==
  CAN_fbk : Inport
  input bus for manual CAN commands1 : BusSelector  OutputSignals=AV_mode_active,gear_fbk,torque_fbk,brake_fbk,steer_fbk
  tag scope: AV_mode_active=global, brake_fbk=global, gear_fbk=global, steer_fbk=global, torque_fbk=global
  wires:
  input bus for manual CAN commands1/2 -> [gear_fbk]  "<gear_fbk>"
  input bus for manual CAN commands1/1 -> [AV_mode_active]  "<AV_mode_active>"
  CAN_fbk/1 -> input bus for manual CAN commands1/1
  input bus for manual CAN commands1/5 -> [steer_fbk]  "<steer_fbk>"
  input bus for manual CAN commands1/4 -> [brake_fbk]  "<brake_fbk>"
  input bus for manual CAN commands1/3 -> [torque_fbk]  "<torque_fbk>"

== system VC_v1p1/Vehicle_Controller/Unpack GNSS FBK ==
  GNSS_fbk : Inport
  Bus Selector1 : BusSelector  OutputSignals=eastr (m),northr (m),psi (deg),vr (m/s),alat (m/s/s),along (m/s/s),pitch (rad)
  tag scope: alat=global, along=global, eastr=global, northr=global, pitch=global, psi=global, vcar=global
  wires:
  GNSS_fbk/1 -> Bus Selector1/1
  Bus Selector1/4 -> [vcar]  "<vr (m/s)>"
  Bus Selector1/5 -> [alat]  "<alat (m/s/s)>"
  Bus Selector1/1 -> [eastr]  "<eastr (m)>"
  Bus Selector1/6 -> [along]  "<along (m/s/s)>"
  Bus Selector1/3 -> [psi]  "<psi (deg)>"
  Bus Selector1/2 -> [northr]  "<northr (m)>"
  Bus Selector1/7 -> [pitch]  "<pitch (rad)>"

== system VC_v1p1/Vehicle_Controller/Waypoint Path Analyzer ==
  Waypoint Path Analysis : Subsystem
  tag scope: east_target=global, end_of_data=global, north_target=global, signal_cmd=global, vref=global, wpt_index=global, xterr=global
  wires:
  [eastr] -> Waypoint Path Analysis/3(eastr)
  Waypoint Path Analysis/2(vref) -> [vref]
  [path_mode] -> Waypoint Path Analysis/1(path_mode)
  [par_bus] -> Waypoint Path Analysis/4(par)
  Waypoint Path Analysis/5(signal_cmd) -> [signal_cmd]  "signal_cmd"
  Waypoint Path Analysis/4(east_target) -> [east_target]
  [northr] -> Waypoint Path Analysis/2(northr)
  Waypoint Path Analysis/3(north_target) -> [north_target]
  [WPT_BUS] -> Waypoint Path Analysis/6(WPT_BUS)
  Waypoint Path Analysis/1(wpt_index) -> [wpt_index]
  [wpt_status_change] -> Waypoint Path Analysis/5(wpt_status_change)
  Waypoint Path Analysis/6(xterr) -> [xterr]
  Waypoint Path Analysis/7(end_of_data) -> [end_of_data]
